simulink model "ex6_v1_backup"  (R2016b)
settings: Solver=ode23s  StartTime=0.0  StopTime=0.5  RelTol=1e-3
InitFcn:
  | param
undefined symbols (not defined in the file): A, A1, A2, B, beta, C, Cf1, Cf2, d, D0, df, fe0, m, p1q0, p2q0, Ps, Pt, Rv, smax, vn, vp, vq0, xvq0
libraries: simulink x3
settings Model: Creator=Philipp  LastModifiedBy=Philipp

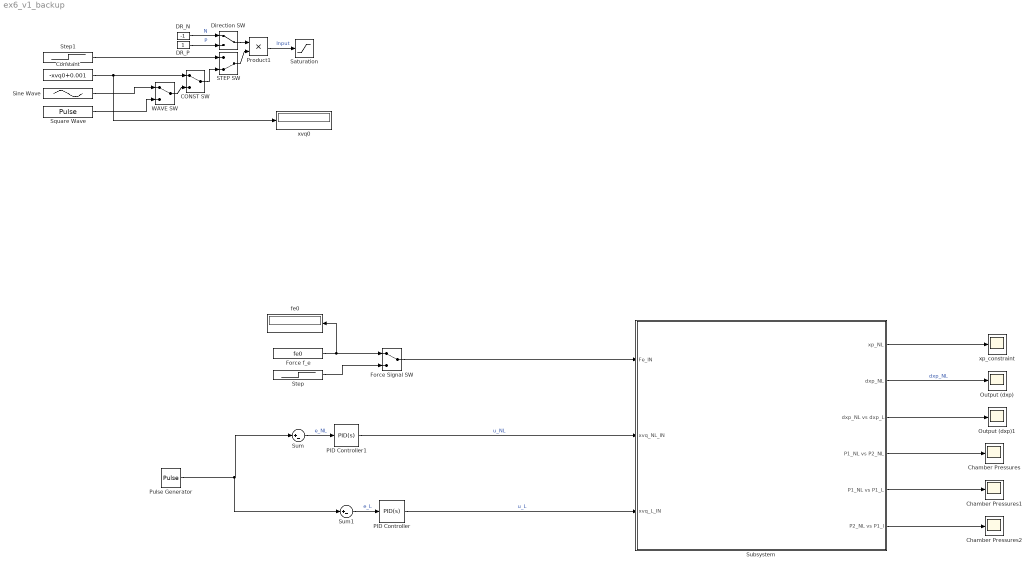
== system ex6_v1_backup ==
  CONST SW : ManualSwitch
  Chamber Pressures : Scope
  Chamber Pressures1 : Scope
  Chamber Pressures2 : Scope
  Constant : Constant  Value=-xvq0+0.001
  DR_N : Constant  Value=-1
  "DR_P " : Constant
  Direction SW : ManualSwitch
  Force Signal SW : ManualSwitch
  Force f_e : Constant  Value=fe0
  Output (dxp) : Scope
  Output (dxp)1 : Scope
  PID Controller : simulink/Continuous/PID Controller  Controller=PID  TimeDomain=Continuous-time  SampleTime=-1  IntegratorMethod=Forward Euler  FilterMethod=Forward Euler  Form=Parallel  UseFilter=on  ControllerParametersSource=internal  P=1  I=1  D=0  N=100  InitialConditionSource=internal  InitialConditionForIntegrator=0  InitialConditionForFilter=0  ExternalReset=none  LimitOutput=off  UpperSaturationLimit=inf  LowerSaturationLimit=-inf  LinearizeAsGain=on  AntiWindupMode=none  Kb=1  TrackingMode=off  Kt=1  PParamMin=[]  PParamMax=[]  IParamMin=[]  IParamMax=[]  DParamMin=[]  DParamMax=[]  NParamMin=[]  NParamMax=[]  KbParamMin=[]  KbParamMax=[]  KtParamMin=[]  KtParamMax=[]  POutMin=[]  POutMax=[]  IOutMin=[]  IOutMax=[]  DOutMin=[]  DOutMax=[]  NOutMin=[]  NOutMax=[]  KbOutMin=[]  KbOutMax=[]  KtOutMin=[]  KtOutMax=[]  IntegratorOutMin=[]  IntegratorOutMax=[]  FilterOutMin=[]  FilterOutMax=[]  SumOutMin=[]  SumOutMax=[]  SumI1OutMin=[]  SumI1OutMax=[]  SumI2OutMin=[]  SumI2OutMax=[]  SumI3OutMin=[]  SumI3OutMax=[]  SumDOutMin=[]  SumDOutMax=[]  SaturationOutMin=[]  SaturationOutMax=[]  IntegratorContinuousStateAttributes=''  IntegratorStateMustResolveToSignalObject=off  IntegratorRTWStateStorageClass=Auto  FilterContinuousStateAttributes=''  FilterStateMustResolveToSignalObject=off  FilterRTWStateStorageClass=Auto  DifferentiatorICPrevScaledInput=0  DifferentiatorOutMin=[]  DifferentiatorOutMax=[]
  PID Controller1 : simulink/Continuous/PID Controller  Controller=PID  TimeDomain=Continuous-time  SampleTime=-1  IntegratorMethod=Forward Euler  FilterMethod=Forward Euler  Form=Parallel  UseFilter=on  ControllerParametersSource=internal  P=1  I=1  D=0  N=100  InitialConditionSource=internal  InitialConditionForIntegrator=0  InitialConditionForFilter=0  ExternalReset=none  LimitOutput=off  UpperSaturationLimit=inf  LowerSaturationLimit=-inf  LinearizeAsGain=on  AntiWindupMode=none  Kb=1  TrackingMode=off  Kt=1  PParamMin=[]  PParamMax=[]  IParamMin=[]  IParamMax=[]  DParamMin=[]  DParamMax=[]  NParamMin=[]  NParamMax=[]  KbParamMin=[]  KbParamMax=[]  KtParamMin=[]  KtParamMax=[]  POutMin=[]  POutMax=[]  IOutMin=[]  IOutMax=[]  DOutMin=[]  DOutMax=[]  NOutMin=[]  NOutMax=[]  KbOutMin=[]  KbOutMax=[]  KtOutMin=[]  KtOutMax=[]  IntegratorOutMin=[]  IntegratorOutMax=[]  FilterOutMin=[]  FilterOutMax=[]  SumOutMin=[]  SumOutMax=[]  SumI1OutMin=[]  SumI1OutMax=[]  SumI2OutMin=[]  SumI2OutMax=[]  SumI3OutMin=[]  SumI3OutMax=[]  SumDOutMin=[]  SumDOutMax=[]  SaturationOutMin=[]  SaturationOutMax=[]  IntegratorContinuousStateAttributes=''  IntegratorStateMustResolveToSignalObject=off  IntegratorRTWStateStorageClass=Auto  FilterContinuousStateAttributes=''  FilterStateMustResolveToSignalObject=off  FilterRTWStateStorageClass=Auto  DifferentiatorICPrevScaledInput=0  DifferentiatorOutMin=[]  DifferentiatorOutMax=[]
  Product1 : Product
  Pulse Generator : DiscretePulseGenerator  PulseType=Time based  Amplitude=0.3  Period=0.5  PulseWidth=5
  STEP SW : ManualSwitch  CurrentSetting=0
  Saturation : Saturate  UpperLimit=vp  LowerLimit=vn
  Sine Wave : Sin  Amplitude=xvq0  Frequency=2*pi*1/2  Phase=pi/2  SampleTime=0
  Square Wave : DiscretePulseGenerator  PulseType=Time based  Amplitude=0.0001  PulseWidth=50
  Step : Step  Time=0.12  After=0  SampleTime=0
  Step1 : Step  Time=0  After=0.005  SampleTime=0
  Subsystem : Subsystem
  Sum : Sum  Inputs=|+-
  Sum1 : Sum  Inputs=|+-
  WAVE SW : ManualSwitch
  fe0 : Display
  xp_constraint : Scope
  xvq0 : Display
  wires:
  Product1/1 -> Saturation/1  "Input"
  Direction SW/1 -> Product1/1
  DR_N/1 -> Direction SW/1  "N"
  "DR_P "/1 -> Direction SW/2  "P"
  Force f_e/1 -> Force Signal SW/1, fe0/1
  Step/1 -> Force Signal SW/2
  Sine Wave/1 -> WAVE SW/1
  WAVE SW/1 -> CONST SW/2
  Square Wave/1 -> WAVE SW/2
  CONST SW/1 -> STEP SW/2
  Step1/1 -> STEP SW/1
  STEP SW/1 -> Product1/2
  Constant/1 -> xvq0/1, CONST SW/1
  Force Signal SW/1 -> Subsystem/1(Fe_IN)
  Subsystem/1(xp_NL) -> xp_constraint/1
  Subsystem/2(dxp_NL) -> Output (dxp)/1  "dxp_NL"
  Subsystem/3(dxp_NL vs dxp_L) -> Output (dxp)1/1
  Subsystem/4(P1_NL vs P2_NL) -> Chamber Pressures/1
  Subsystem/5(P1_NL vs P1_L) -> Chamber Pressures1/1
  Subsystem/6(P2_NL vs P1_l) -> Chamber Pressures2/1
  PID Controller/1 -> Subsystem/3(xvq_L_IN)  "u_L"
  Sum1/1 -> PID Controller/1  "e_L"
  ? -> Sum1/2  "dxp_L"
  Sum/1 -> PID Controller1/1  "e_NL"
  PID Controller1/1 -> Subsystem/2(xvq_NL_IN)  "u_NL"
  Pulse Generator/1 -> Sum1/1, Sum/1
  ? -> Sum/2

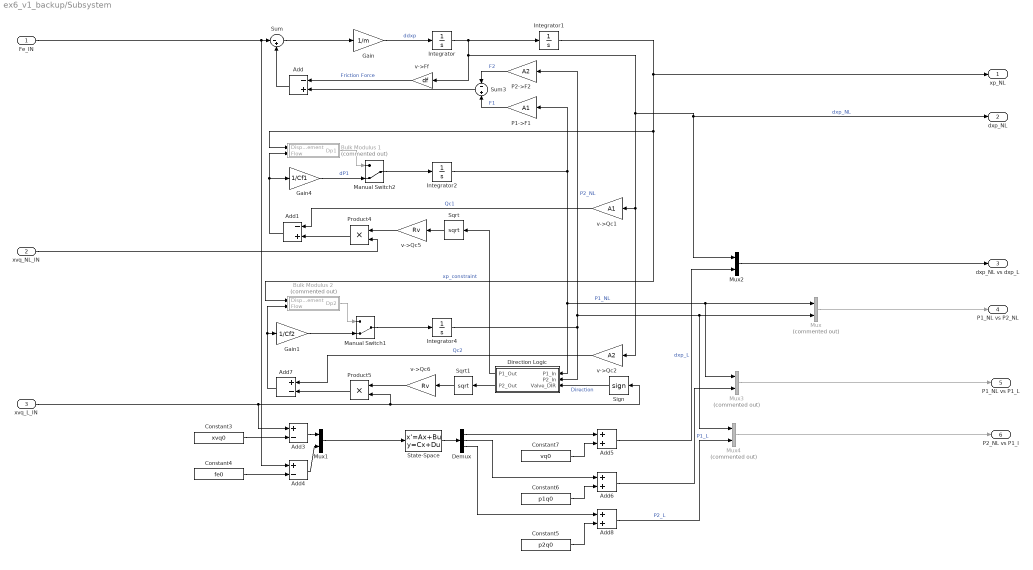
== system ex6_v1_backup/Subsystem ==
  Fe_IN : Inport
  xvq_NL_IN : Inport  Port=2
  xvq_L_IN : Inport  Port=3
  Add : Sum  Inputs=-+
  Add1 : Sum  Inputs=-+
  Add3 : Sum  Inputs=+-
  Add4 : Sum  Inputs=+-
  Add5 : Sum
  Add6 : Sum
  Add7 : Sum  Inputs=+-
  Add8 : Sum
  Bulk Modulus 1 : Subsystem  Commented=on
  Bulk Modulus 2 : Subsystem  Commented=on
  Constant3 : Constant  Value=xvq0
  Constant4 : Constant  Value=fe0
  Constant5 : Constant  Value=p2q0
  Constant6 : Constant  Value=p1q0
  Constant7 : Constant  Value=vq0
  Demux : Demux  Outputs=3
  Direction Logic : Subsystem
  Gain : Gain  Gain=1/m
  Gain1 : Gain  Gain=1/Cf2
  Gain4 : Gain  Gain=1/Cf1
  Integrator : Integrator
  Integrator1 : Integrator  LimitOutput=on  UpperSaturationLimit=(smax/2-d)  LowerSaturationLimit=-(smax/2-d)
  Integrator2 : Integrator
  Integrator4 : Integrator
  Manual Switch1 : ManualSwitch  CurrentSetting=0
  Manual Switch2 : ManualSwitch  CurrentSetting=0
  Mux : Mux  Commented=on  Inputs=2
  Mux1 : Mux  Inputs=2
  Mux2 : Mux  Inputs=2
  Mux3 : Mux  Commented=on  Inputs=2
  Mux4 : Mux  Commented=on  Inputs=2
  P1->F1 : Gain  Gain=A1
  P2->F2 : Gain  Gain=A2
  Product4 : Product
  Product5 : Product
  Sign : Signum
  Sqrt : Sqrt  SaturateOnIntegerOverflow=on
  Sqrt1 : Sqrt  SaturateOnIntegerOverflow=on
  State-Space : StateSpace  A=A  B=B  C=C  D=D0  X0=0
  Sum : Sum  Inputs=|-+
  Sum3 : Sum  Inputs=-+
  v->Ff : Gain  Gain=df
  v->Qc1 : Gain  Gain=A1
  v->Qc2 : Gain  Gain=A2
  v->Qc5 : Gain  Gain=Rv
  v->Qc6 : Gain  Gain=Rv
  xp_NL : Outport
  dxp_NL : Outport  Port=2
  dxp_NL vs dxp_L : Outport  Port=3
  P1_NL vs P2_NL : Outport  Port=4
  P1_NL vs P1_L : Outport  Port=5
  P2_NL vs P1_l : Outport  Port=6
  wires:
  P1->F1/1 -> Sum3/2  "F1"
  P2->F2/1 -> Sum3/1  "F2"
  Sum/1 -> Gain/1
  Add7/1 -> Bulk Modulus 2/2(Flow), Gain1/1
  Integrator4/1 -> Mux/2, Mux4/1, P2->F2/1, Direction Logic/2(P2_In)  "P2_NL"
  Sign/1 -> Direction Logic/3(Valve_DIR)  "Direction"
  Sum3/1 -> Add/2
  Integrator2/1 -> Direction Logic/1(P1_In), Mux/1, Mux3/1, P1->F1/1  "P1_NL"
  Manual Switch1/1 -> Integrator4/1
  v->Qc5/1 -> Product4/1
  Bulk Modulus 1/1(Dp1) -> Manual Switch2/1
  Add/1 -> Sum/2
  Add1/1 -> Bulk Modulus 1/2(Flow), Gain4/1
  Product4/1 -> Add1/2
  Direction Logic/1(P1_Out) -> Sqrt/1
  v->Qc2/1 -> Add7/1  "Qc2"
  Sqrt/1 -> v->Qc5/1
  Sqrt1/1 -> v->Qc6/1
  v->Ff/1 -> Add/1  "Friction Force"
  Direction Logic/2(P2_Out) -> Sqrt1/1
  Gain4/1 -> Manual Switch2/2  "dP1"
  Integrator1/1 -> xp_NL/1, Bulk Modulus 2/1(Displacement), Bulk Modulus 1/1(Displacement)  "xp_constraint"
  Bulk Modulus 2/1(Dp2) -> Manual Switch1/1
  Gain/1 -> Integrator/1  "ddxp"
  Gain1/1 -> Manual Switch1/2
  Mux/1 -> P1_NL vs P2_NL/1
  Product5/1 -> Add7/2
  v->Qc6/1 -> Product5/1
  v->Qc1/1 -> Add1/1  "Qc1"
  Manual Switch2/1 -> Integrator2/1
  Add4/1 -> Mux1/2
  Add8/1 -> Mux4/2  "P2_L"
  Constant4/1 -> Add4/2
  Mux4/1 -> P2_NL vs P1_l/1
  Integrator/1 -> Integrator1/1, v->Qc2/1, v->Qc1/1, dxp_NL/1, Mux2/1, v->Ff/1  "dxp_NL"
  xvq_L_IN/1 -> Sign/1, Product5/2, Add3/1
  Mux2/1 -> dxp_NL vs dxp_L/1
  Constant6/1 -> Add6/2
  Demux/1 -> Add5/1
  Demux/2 -> Add6/1
  Add5/1 -> Mux2/2  "dxp_L"
  Mux1/1 -> State-Space/1
  Mux3/1 -> P1_NL vs P1_L/1
  Add3/1 -> Mux1/1
  Constant3/1 -> Add3/2
  Constant7/1 -> Add5/2
  Fe_IN/1 -> Add4/1, Sum/1
  Constant5/1 -> Add8/2
  Demux/3 -> Add8/1
  Add6/1 -> Mux3/2  "P1_L"
  State-Space/1 -> Demux/1
  xvq_NL_IN/1 -> Product4/2

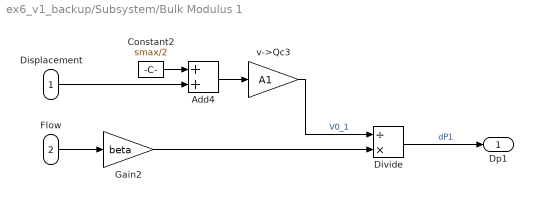
== system ex6_v1_backup/Subsystem/Bulk Modulus 1 ==
  Displacement : Inport
  Flow : Inport  Port=2
  Add4 : Sum
  Constant2 : Constant  Value=smax/2
  Divide : Product  Inputs=/*
  Gain2 : Gain  Gain=beta
  v->Qc3 : Gain  Gain=A1
  Dp1 : Outport
  wires:
  Flow/1 -> Gain2/1
  Displacement/1 -> Add4/2
  Constant2/1 -> Add4/1
  Divide/1 -> Dp1/1  "dP1"
  v->Qc3/1 -> Divide/1  "V0_1"
  Gain2/1 -> Divide/2
  Add4/1 -> v->Qc3/1

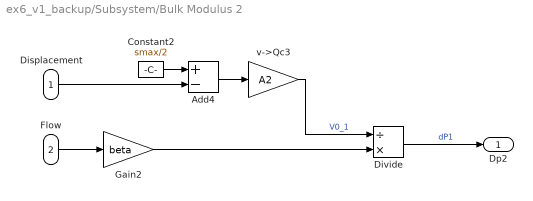
== system ex6_v1_backup/Subsystem/Bulk Modulus 2 ==
  Displacement : Inport
  Flow : Inport  Port=2
  Add4 : Sum  Inputs=+-
  Constant2 : Constant  Value=smax/2
  Divide : Product  Inputs=/*
  Gain2 : Gain  Gain=beta
  v->Qc3 : Gain  Gain=A2
  Dp2 : Outport
  wires:
  Flow/1 -> Gain2/1
  Displacement/1 -> Add4/2
  Constant2/1 -> Add4/1
  Divide/1 -> Dp2/1  "dP1"
  v->Qc3/1 -> Divide/1  "V0_1"
  Gain2/1 -> Divide/2
  Add4/1 -> v->Qc3/1

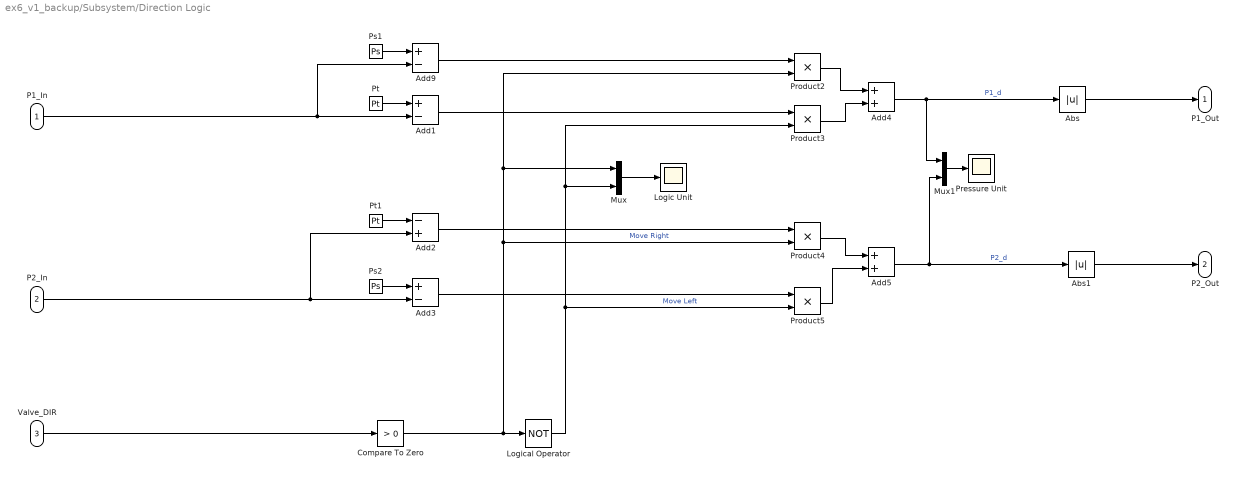
== system ex6_v1_backup/Subsystem/Direction Logic ==
  P1_In : Inport
  P2_In : Inport  Port=2
  Valve_DIR : Inport  Port=3
  Abs : Abs  ZeroCross=off
  Abs1 : Abs
  Add1 : Sum  Inputs=+-
  Add2 : Sum  Inputs=-+
  Add3 : Sum  Inputs=+-
  Add4 : Sum
  Add5 : Sum
  Add9 : Sum  Inputs=+-
  Compare To Zero : simulink/Logic and Bit Operations/Compare To Zero  relop=>  OutDataTypeStr=boolean
  Logic Unit : Scope
  Logical Operator : Logic  Operator=NOT  AllPortsSameDT=off  OutDataTypeStr=boolean
  Mux : Mux  Inputs=2
  Mux1 : Mux  Inputs=2
  Pressure Unit : Scope
  Product{2..5} (4 alike) : Product
  Ps1 : Constant  Value=Ps
  Ps2 : Constant  Value=Ps
  Pt : Constant  Value=Pt
  Pt1 : Constant  Value=Pt
  P1_Out : Outport
  P2_Out : Outport  Port=2
  wires:
  Valve_DIR/1 -> Compare To Zero/1
  Compare To Zero/1 -> Mux/1, Product2/2, Product4/2, Logical Operator/1  "Move Right"
  Logical Operator/1 -> Mux/2, Product3/2, Product5/2  "Move Left"
  Add9/1 -> Product2/1
  Ps1/1 -> Add9/1
  P1_In/1 -> Add1/2, Add9/2
  Add1/1 -> Product3/1
  Add3/1 -> Product5/1
  Ps2/1 -> Add3/1
  P2_In/1 -> Add2/2, Add3/2
  Add2/1 -> Product4/1
  Pt1/1 -> Add2/1
  Pt/1 -> Add1/1
  Product2/1 -> Add4/1
  Product3/1 -> Add4/2
  Product4/1 -> Add5/1
  Product5/1 -> Add5/2
  Add4/1 -> Abs/1, Mux1/1  "P1_d"
  Abs/1 -> P1_Out/1
  Abs1/1 -> P2_Out/1
  Add5/1 -> Abs1/1, Mux1/2  "P2_d"
  Mux/1 -> Logic Unit/1
  Mux1/1 -> Pressure Unit/1
